simulink model "Wheelspeed_Logik_15_01_26"  (R2025b)
settings: Solver=ode1  StartTime=0.0  StopTime=10.0  FixedStep=0.0001  RelTol=1e-3
libraries: simulink x1
settings Model: Creator=finneinhoff  LastModifiedBy=finneinhoff

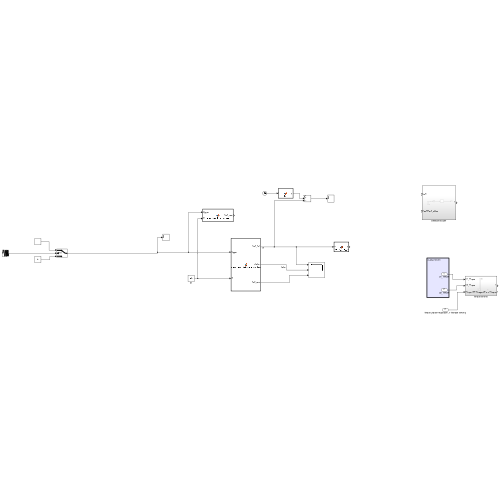
[thumbnail: Simulink's stored preview of the top-level diagram]
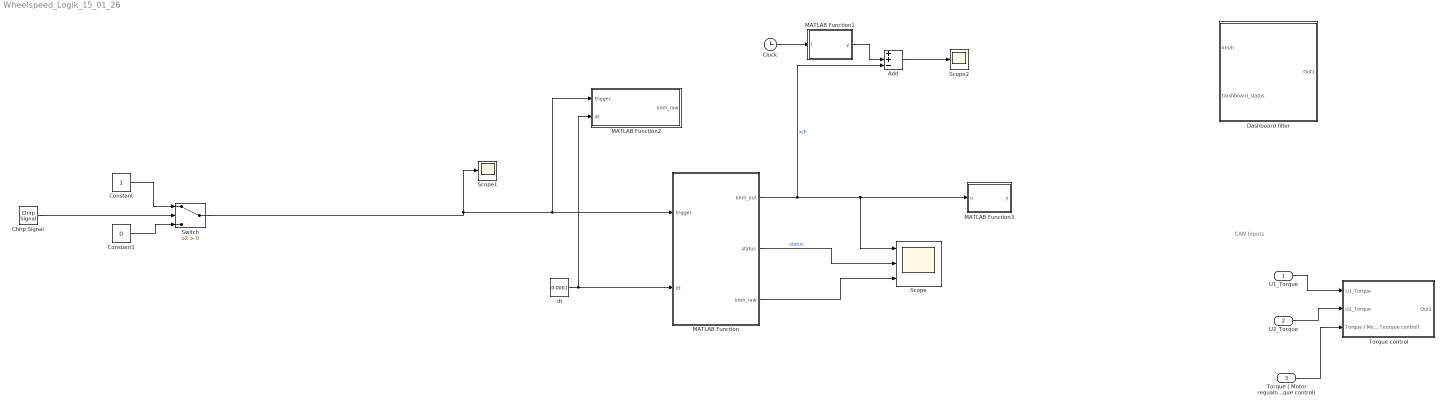
== system Wheelspeed_Logik_15_01_26 ==
  note: CAN Inputs
  U1_Torque : Inport
  U2_Torque : Inport  Port=2
  "Torque ( Motor regualtion -> Tourque control)" : Inport  Port=3
  Add : Sum  Inputs=++-
  Chirp Signal : simulink/Sources/Chirp Signal  f1=1  T=10  f2=1800
  Clock : Clock
  Constant : Constant
  Constant1 : Constant  Value=0
  Dashboard filter : Subsystem
  MATLAB Function : MATLAB Function  TreatAsAtomicUnit=on
  MATLAB Function1 : MATLAB Function  TreatAsAtomicUnit=on
  MATLAB Function2 : MATLAB Function  TreatAsAtomicUnit=on
  MATLAB Function3 : MATLAB Function  TreatAsAtomicUnit=on
  Scope : Scope  NumInputPorts=3
      settings: ActiveDisplayYMinimum=-26.004496664270235  ActiveDisplayYMaximum=234.04046997843218
  Scope1 : Scope
      settings: ActiveDisplayYMinimum=-0.21801651491494711  ActiveDisplayYMaximum=1.2439728540304662
  Scope2 : Scope
      settings: ActiveDisplayYMinimum=-1  ActiveDisplayYMaximum=1  DataLoggingVariableName=ScopeData2
  Switch : Switch  Criteria=u2 > Threshold  OutDataTypeStr=double  SaturateOnIntegerOverflow=off  InputSameDT=off
  Torque control : Subsystem
  dt : Constant  Value=0.0001
  wires:
  dt/1 -> MATLAB Function/2(dt), MATLAB Function2/2(dt)
  Constant/1 -> Switch/1
  Constant1/1 -> Switch/3
  MATLAB Function/2(status) -> Scope/2  "status"
  Chirp Signal/1 -> Switch/2
  MATLAB Function/1(kmh_out) -> MATLAB Function3/1(u), Scope/1, Add/3  "k/h"
  Clock/1 -> MATLAB Function1/1(t)
  MATLAB Function1/1(y) -> Add/2
  Add/1 -> Scope2/1
  U1_Torque/1 -> Torque control/1(U1_Torque)
  U2_Torque/1 -> Torque control/2(U2_Torque)
  "Torque ( Motor regualtion -> Tourque control)"/1 -> Torque control/3("Torque ( Motor regualtion -> Tourque control)")
  MATLAB Function/3(kmh_raw) -> Scope/3
  Switch/1 -> Scope1/1, MATLAB Function2/1(trigger), MATLAB Function/1(trigger)

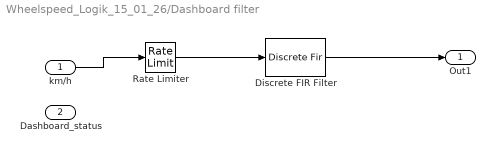
== system Wheelspeed_Logik_15_01_26/Dashboard filter ==
  km/h : Inport
  Dashboard_status : Inport  Port=2
  Discrete FIR Filter : DiscreteFir
  Rate Limiter : RateLimiter  SampleTimeMode=inherited
  Out1 : Outport
  wires:
  km/h/1 -> Rate Limiter/1
  Rate Limiter/1 -> Discrete FIR Filter/1
  Discrete FIR Filter/1 -> Out1/1

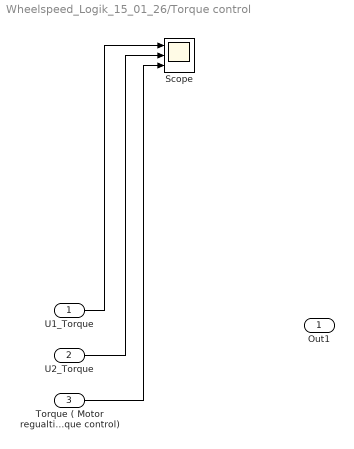
== system Wheelspeed_Logik_15_01_26/Torque control ==
  U1_Torque : Inport
  U2_Torque : Inport  Port=2
  "Torque ( Motor regualtion -> Tourque control)" : Inport  Port=3
  Scope : Scope  NumInputPorts=3
      settings: DataLoggingVariableName=ScopeData3
  Out1 : Outport
  wires:
  U1_Torque/1 -> Scope/1
  U2_Torque/1 -> Scope/2
  "Torque ( Motor regualtion -> Tourque control)"/1 -> Scope/3

== matlab function Wheelspeed_Logik_15_01_26/MATLAB Function1 ==
  data: t input; y output
function y = fcn(t)
    % t ist die aktuelle Simulationszeit (muss von außen kommen)

    % 1. Berechnung von u (Rampe)
    % Steigung = 1800 / 10s = 180 pro Sekunde
    rate = 180;
    
    if t <= 10
        u = rate * t;       % Linearer Anstieg
    else
        u = 1800;           % Begrenzung auf 1800 nach 10s
    end

    % 2. Deine eigentliche Berechnung mit u
    % (Punkte statt Kommas!)
    y = (u * 1.6 * 3.6) / 50;
    
end

== matlab function Wheelspeed_Logik_15_01_26/MATLAB Function ==
  data: trigger input; kmh_out output; dt input; status output; kmh_raw output
function [kmh_out, status, kmh_raw] = wheelspeed_fs2026_immediate(trigger, dt)
    
    % --- PARAMETER ---
    teeth  = 50;
    circum = 1.6;
    
    DEBOUNCE_TIME = 0.0001; 
    
    % Maximale Geschwindigkeitbeim Kaltstart 
    MAX_STARTUP_KMH = 5; 
    
    % Frequenz-Grenzen & Filter
    FREQ_FAST = 300;   
    FREQ_SLOW = 1200;  
    TAU_FAST  = 0.01; 
    TAU_SLOW  = 0.01; 
    
    % --- SPEICHER ---
    persistent timer;
    persistent v_smooth;
    persistent prev_trigger;
    persistent v_buffer; 
    persistent first_run;
    persistent raw_hold;
    
    % --- INIT ---
    if isempty(timer)
        timer = 0;
        v_smooth = 0;
        prev_trigger = 0;
        v_buffer = [0, 0, 0, 0, 0]; 
        first_run = true;
        raw_hold = 0;
    end
    
    % Default Output
    kmh_out = v_smooth * 3.6;
    kmh_raw = raw_hold * 3.6;
 
    % Timer Update
    timer = timer + dt;
    status = 0; 
    
    % Flanke
    is_rising = (trigger >= 1) && (prev_trigger < 1);
    prev_trigger = trigger;
    
    
    % MESSUNG
    if is_rising
        
        % 1. Debounce
        if timer < DEBOUNCE_TIME
            return; 
        end 
        
        % 2. Roh-Messung
        current_period = timer;
        timer = 0; 
        
        dist_per_tooth = circum / teeth;
        v_raw_ms = dist_per_tooth / current_period;
        raw_hold = v_raw_ms;
        kmh_raw = raw_hold * 3.6;

        %  ÄNDERUNG ERSTER ZAHN WIRD AKZEPTIERT
        if first_run
            % Wir begrenzen den allerersten Wert auf MAX_STARTUP_KMH.
            % lässt
            % echte Geschwindigkeiten sofort durch.
            
            v_startup = v_raw_ms;
            max_ms = MAX_STARTUP_KMH / 3.6;

            if v_startup > max_ms
                v_startup = max_ms; % Kappen auf 300 km/h
            end
            raw_hold = v_startup;
            % Buffer & Output sofort setzen
            v_buffer(:) = v_startup;
            v_smooth = v_startup;
            kmh_out = v_smooth * 3.6;
            
            first_run = false;
            status = 1;
            return; 
        end
        
        
        % 3. Normaler Betrieb (Ab Zahn 2)
        v_buffer(1) = v_buffer(2);
        v_buffer(2) = v_buffer(3);
        v_buffer(3) = v_buffer(4);
        v_buffer(4) = v_buffer(5);
        v_buffer(5) = v_raw_ms;
        
        % Adaptive Logik
        freq_hz = 1.0 / current_period;
        v_target = 0;    
        current_tau = 0;  
        
        if freq_hz < FREQ_FAST
            sorted = sort(v_buffer);
            v_target = sorted(3); 
            current_tau = TAU_FAST;
        elseif freq_hz > FREQ_SLOW
            v_target = v_raw_ms;  
            current_tau = TAU_SLOW;
        else
            factor = (freq_hz - FREQ_FAST) / (FREQ_SLOW - FREQ_FAST);
            current_tau = TAU_FAST + factor * (TAU_SLOW - TAU_FAST);
            v_target = v_raw_ms; 
        end
        
        % Filter
        alpha = current_period / (current_tau + current_period);
        v_smooth = v_smooth + alpha * (v_target - v_smooth);
        
        status = 1; 
        kmh_out = v_smooth * 3.6;
        
    end 
    
    
    % TIMEOUT
    if (v_smooth < 10.0) && (v_smooth > 0.1)
        expected_period = (circum / teeth) / v_smooth; % v_smooth ist m/s
        
        if timer > (expected_period * 3.0)
            alpha_decay = dt / TAU_FAST; 
            v_smooth = v_smooth * (1 - alpha_decay);
            kmh_out = v_smooth * 3.6;
        end
    end 
    
    % Stillstand
    if timer > 0.5
        v_smooth = 0;
        raw_hold = 0;
        status = 3;
        kmh_out = 0;
    end

end

== matlab function Wheelspeed_Logik_15_01_26/MATLAB Function2 ==
  data: trigger input; kmh_raw output; dt input
function kmh_raw = wheelspeed_raw_simple(trigger, dt)
    
    % --- KONSTANTEN ---
    teeth  = 50;        % Anzahl Zähne
    circum = 1.6;       % Radumfang in Metern
    
    % --- GEDÄCHTNIS (Persistent) ---
    persistent timer;        % Die Stoppuhr
    persistent prev_trigger; % Vorheriger Sensorzustand
    persistent last_kmh;     % Letzter berechneter Wert
    
    % Beim allerersten Start alles nullen
    if isempty(timer)
        timer = 0;
        prev_trigger = 0;
        last_kmh = 0;
    end
    
    % 1. Zeit weiterlaufen lassen
    timer = timer + dt;
    
    % 2. Flanke erkennen (Zahn kommt vorbei)
    is_rising = (trigger >= 1) && (prev_trigger < 1);
    prev_trigger = trigger; % Fürs nächste Mal merken
    
    % 3. BERECHNUNG (Nur wenn ein Zahn da ist)
    if is_rising
        
        % Die einfache Physik-Formel: v = s / t
        
        strecke_pro_zahn = circum / teeth;  % s (Weg)
        zeit_seit_letztem_zahn = timer;     % t (Zeit)
        
        if zeit_seit_letztem_zahn > 0 % Schutz vor Division durch Null
            v_ms = strecke_pro_zahn / zeit_seit_letztem_zahn;
            
            % Umrechnung in km/h und speichern
            last_kmh = v_ms * 3.6;
        end
        
        % Stoppuhr resetten für den nächsten Zahn
        timer = 0;
    end
    
    % --- NOT-AUS (Timeout) ---
    % Ohne das hier würde der Tacho beim Anhalten für immer 
    % auf dem letzten Wert (z.B. 50 km/h) stehen bleiben.
    if timer > 0.5
        last_kmh = 0;
    end
    
    % Ausgabe
    kmh_raw = last_kmh;
    
end

== matlab function Wheelspeed_Logik_15_01_26/MATLAB Function3 ==
  data: u input; y output
function y = median_filter_fifo(u)
    % persistent speichert die Variable zwischen den Zeitschritten
    persistent buffer
    
    % Initialisierung: Beim ersten Start den Buffer mit dem ersten Wert füllen
    if isempty(buffer)
        buffer = [u; u; u; u; u;u;u;u;u]; % 5-Werte Buffer vollmachen
    end
    
    % FIFO Prinzip (First In, First Out)
    % Wir setzen den neuen Wert oben drauf und löschen den ältesten (den letzten)
    buffer = [u; buffer(1:8)];
    
    % Median berechnen (sortiert intern und nimmt die Mitte)
    y = median(buffer);
end
